simulink model "BEncoderError"  (R2024b)
settings: Solver=FixedStepDiscrete  StartTime=0.0  StopTime=10.0  FixedStep=0.001  RelTol=1e-3  SampleTimeConstraint=STIndependent
libraries: simulink x8
settings Model: DataDictionary=Master_Dictionary.sldd  EnableAccessToBaseWorkspace=off  Creator=torni  LastModifiedBy=will
settings SolverCC: AlgebraicLoopSolver=TrustRegion
settings DataIOCC: ReturnWorkspaceOutputs=off
settings OptimizationCC: DefaultParameterBehavior=Inlined  EnhancedBackFolding=on  PassReuseOutputArgsAs=Individual arguments  ZeroExternalMemoryAtStartup=off  ZeroInternalMemoryAtStartup=off  OptimizeBlockOrder=speed  DifferentSizesBufferReuse=on  OptimizationCustomize=off  EfficientTunableParamExpr=on
settings DebuggingCC: ParameterTunabilityLossMsg=error  UnconnectedInputMsg=warning  UnconnectedOutputMsg=warning  UnconnectedLineMsg=warning  ArithmeticOperatorsInVariantConditions=warning
settings HardwareCC: TargetLargestAtomicInteger=Long  TargetLargestAtomicFloat=Double  TargetIntDivRoundTo=Zero  TargetEndianess=LittleEndian  TargetHWDeviceType=ARM Compatible->ARM Cortex-M  ProdEqTarget=off
settings ModelReferenceCC: EnableRefExpFcnMdlSchedulingChecks=on
settings SFSimCC: MATLABDynamicMemAlloc=off  CustomCodeUndefinedFunction=UseInterfaceOnly
settings RTWCC: Description=Embedded Coder  SystemTargetFile=ert.tlc  TemplateMakefile=ert_default_tmf  Toolchain=GNU Tools for ARM Embedded Processors  RTWCompilerOptimization=on  GPUComputeCapability=3.5
settings CodeAppCC: ForceParamTrailComments=on  IgnoreCustomStorageClasses=off  OperatorAnnotations=on  SimulinkDataObjDesc=on  SFDataObjDesc=on  InsertBlockDesc=on
settings ERTTargetCC: TargetLangStandard=C99 (ISO)  GenerateSampleERTMain=on  ERTCustomFileTemplate=example_file_process.tlc

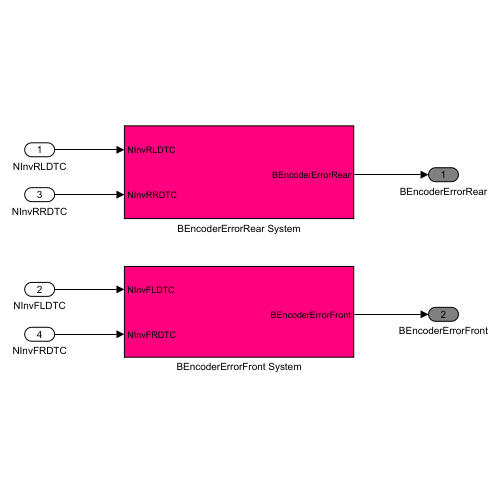
[thumbnail: Simulink's stored preview of the top-level diagram]
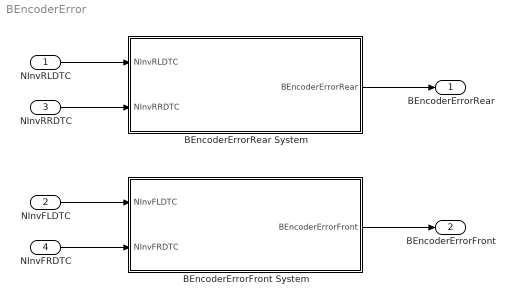
== system BEncoderError ==
  NInvRLDTC : Inport  OutDataTypeStr=double
  NInvFLDTC : Inport  Port=2  OutDataTypeStr=double
  NInvRRDTC : Inport  Port=3  OutDataTypeStr=double
  NInvFRDTC : Inport  Port=4  OutDataTypeStr=double
  BEncoderErrorFront System : Subsystem
  BEncoderErrorRear System : Subsystem
  BEncoderErrorRear : Outport  OutDataTypeStr=boolean  VectorParamsAs1DForOutWhenUnconnected=off
  BEncoderErrorFront : Outport  Port=2  OutDataTypeStr=boolean  VectorParamsAs1DForOutWhenUnconnected=off
  wires:
  BEncoderErrorFront System/1(BEncoderErrorFront) -> BEncoderErrorFront/1
  NInvRRDTC/1 -> BEncoderErrorRear System/2(NInvRRDTC)
  NInvFLDTC/1 -> BEncoderErrorFront System/1(NInvFLDTC)
  BEncoderErrorRear System/1(BEncoderErrorRear) -> BEncoderErrorRear/1
  NInvFRDTC/1 -> BEncoderErrorFront System/2(NInvFRDTC)
  NInvRLDTC/1 -> BEncoderErrorRear System/1(NInvRLDTC)

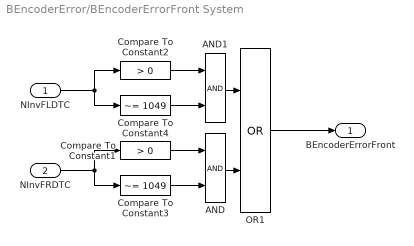
== system BEncoderError/BEncoderErrorFront System ==
  NInvFLDTC : Inport  OutDataTypeStr=double
  NInvFRDTC : Inport  Port=2  OutDataTypeStr=double
  AND : Logic  AllPortsSameDT=off  OutDataTypeStr=boolean
  AND1 : Logic  AllPortsSameDT=off  OutDataTypeStr=boolean
  Compare To Constant1 : simulink/Logic and Bit Operations/Compare To Constant  relop=>  const=0  OutDataTypeStr=boolean
  Compare To Constant2 : simulink/Logic and Bit Operations/Compare To Constant  relop=>  const=0  OutDataTypeStr=boolean
  Compare To Constant3 : simulink/Logic and Bit Operations/Compare To Constant  relop=~=  const=1049  OutDataTypeStr=boolean
  Compare To Constant4 : simulink/Logic and Bit Operations/Compare To Constant  relop=~=  const=1049  OutDataTypeStr=boolean
  OR1 : Logic  Operator=OR  AllPortsSameDT=off  OutDataTypeStr=boolean
  BEncoderErrorFront : Outport  OutDataTypeStr=boolean  VectorParamsAs1DForOutWhenUnconnected=off
  wires:
  OR1/1 -> BEncoderErrorFront/1
  Compare To Constant2/1 -> AND1/1
  Compare To Constant1/1 -> AND/1
  NInvFLDTC/1 -> Compare To Constant2/1, Compare To Constant4/1
  Compare To Constant3/1 -> AND/2
  Compare To Constant4/1 -> AND1/2
  NInvFRDTC/1 -> Compare To Constant3/1, Compare To Constant1/1
  AND1/1 -> OR1/1
  AND/1 -> OR1/2

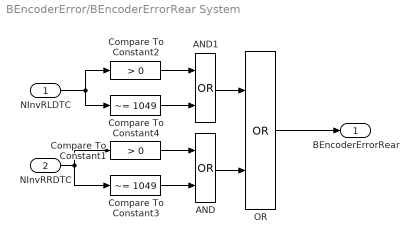
== system BEncoderError/BEncoderErrorRear System ==
  NInvRLDTC : Inport  OutDataTypeStr=double
  NInvRRDTC : Inport  Port=2  OutDataTypeStr=double
  AND : Logic  Operator=OR  AllPortsSameDT=off  OutDataTypeStr=boolean
  AND1 : Logic  Operator=OR  AllPortsSameDT=off  OutDataTypeStr=boolean
  Compare To Constant1 : simulink/Logic and Bit Operations/Compare To Constant  relop=>  const=0  OutDataTypeStr=boolean
  Compare To Constant2 : simulink/Logic and Bit Operations/Compare To Constant  relop=>  const=0  OutDataTypeStr=boolean
  Compare To Constant3 : simulink/Logic and Bit Operations/Compare To Constant  relop=~=  const=1049  OutDataTypeStr=boolean
  Compare To Constant4 : simulink/Logic and Bit Operations/Compare To Constant  relop=~=  const=1049  OutDataTypeStr=boolean
  OR : Logic  Operator=OR  AllPortsSameDT=off  OutDataTypeStr=boolean
  BEncoderErrorRear : Outport  OutDataTypeStr=boolean  VectorParamsAs1DForOutWhenUnconnected=off
  wires:
  OR/1 -> BEncoderErrorRear/1
  AND1/1 -> OR/1
  Compare To Constant3/1 -> AND/2
  AND/1 -> OR/2
  Compare To Constant1/1 -> AND/1
  NInvRRDTC/1 -> Compare To Constant3/1, Compare To Constant1/1
  Compare To Constant2/1 -> AND1/1
  Compare To Constant4/1 -> AND1/2
  NInvRLDTC/1 -> Compare To Constant4/1, Compare To Constant2/1
